simulink library "uavsimBlockset_InstrumentPanel"  (Simulink 8.0)
settings: Solver=ode45  StartTime=0.0  StopTime=10.0  RelTol=1e-3
libraries: aerosimlib x2
settings Model: Creator=mstolle  LastModifiedBy=j.bolting

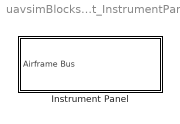
== system uavsimBlockset_InstrumentPanel ==
  Instrument Panel : Subsystem

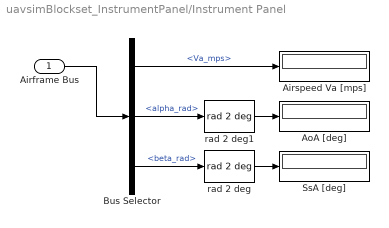
== system uavsimBlockset_InstrumentPanel/Instrument Panel ==
  Airframe Bus : Inport  OutDataTypeStr=Bus: Airframe
  Airspeed Va [mps] : Display
  AoA [deg] : Display
  Bus Selector : BusSelector  OutputSignals=Aero.Va_mps,Aero.alpha_rad,Aero.beta_rad
  SsA [deg] : Display
  rad 2 deg : aerosimlib/Unit Conversion/Angular position/rad 2 deg
  rad 2 deg1 : aerosimlib/Unit Conversion/Angular position/rad 2 deg
  wires:
  Airframe Bus/1 -> Bus Selector/1
  Bus Selector/1 -> Airspeed Va [mps]/1  "<Va_mps>"
  Bus Selector/3 -> rad 2 deg/1  "<beta_rad>"
  Bus Selector/2 -> rad 2 deg1/1  "<alpha_rad>"
  rad 2 deg/1 -> SsA [deg]/1
  rad 2 deg1/1 -> AoA [deg]/1
